simulink model "lab2_floating_01slx"  (R2022a)
settings: Solver=VariableStepAuto  StartTime=0.0  StopTime=10.0  RelTol=1e-3
settings Model: Creator=Illia  LastModifiedBy=Illia

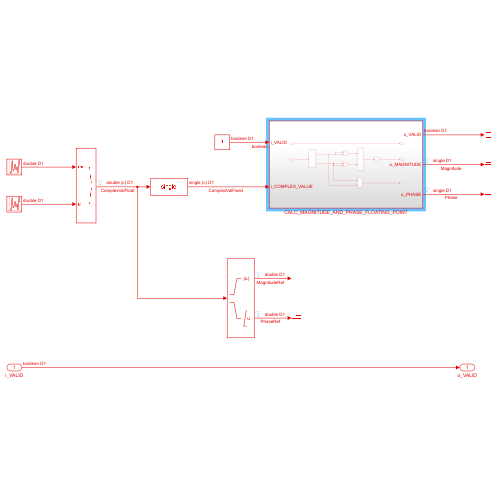
[thumbnail: Simulink's stored preview of the top-level diagram]
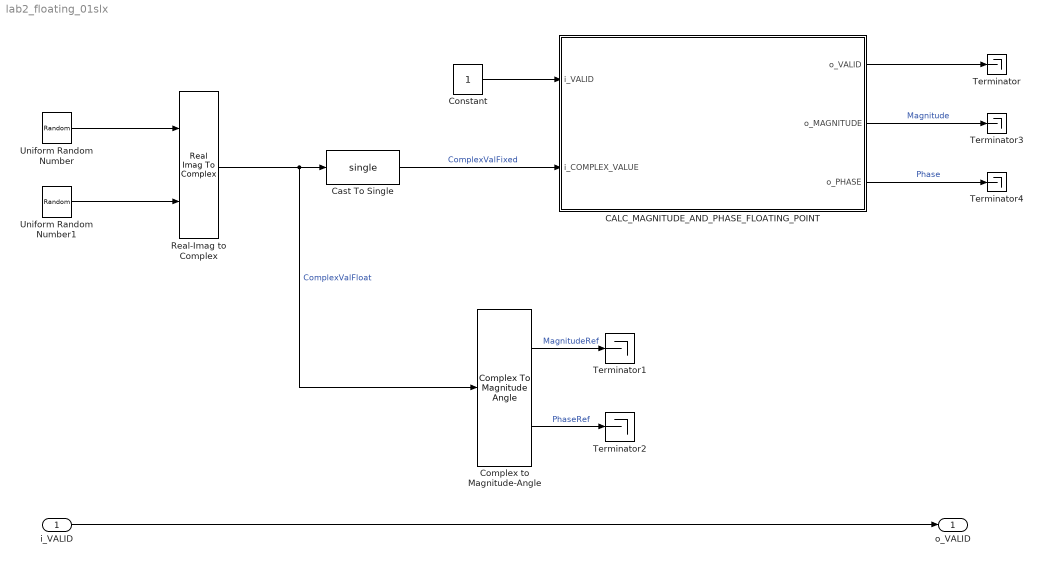
== system lab2_floating_01slx ==
  i_VALID : Inport  OutDataTypeStr=boolean
  CALC_MAGNITUDE_AND_PHASE_FLOATING_POINT : Subsystem
  Cast To Single : DataTypeConversion  OutDataTypeStr=single  RndMeth=Nearest  SaturateOnIntegerOverflow=off
  Complex to Magnitude-Angle : ComplexToMagnitudeAngle
  Constant : Constant  OutDataTypeStr=boolean  SampleTime=1
  Real-Imag to Complex : RealImagToComplex
  Terminator{,1..4} (5 alike) : Terminator
  Uniform Random Number : UniformRandomNumber  Minimum=-4  Maximum=4  Seed=5  SampleTime=1
  Uniform Random Number1 : UniformRandomNumber  Seed=6  SampleTime=1
  o_VALID : Outport  VectorParamsAs1DForOutWhenUnconnected=off
  wires:
  i_VALID/1 -> o_VALID/1
  Cast To Single/1 -> CALC_MAGNITUDE_AND_PHASE_FLOATING_POINT/2(i_COMPLEX_VALUE)  "ComplexValFixed"
  Constant/1 -> CALC_MAGNITUDE_AND_PHASE_FLOATING_POINT/1(i_VALID)
  CALC_MAGNITUDE_AND_PHASE_FLOATING_POINT/3(o_PHASE) -> Terminator4/1  "Phase"
  Complex to Magnitude-Angle/2 -> Terminator2/1  "PhaseRef"
  CALC_MAGNITUDE_AND_PHASE_FLOATING_POINT/2(o_MAGNITUDE) -> Terminator3/1  "Magnitude"
  Real-Imag to Complex/1 -> Cast To Single/1, Complex to Magnitude-Angle/1  "ComplexValFloat"
  Uniform Random Number/1 -> Real-Imag to Complex/1
  Complex to Magnitude-Angle/1 -> Terminator1/1  "MagnitudeRef"
  Uniform Random Number1/1 -> Real-Imag to Complex/2
  CALC_MAGNITUDE_AND_PHASE_FLOATING_POINT/1(o_VALID) -> Terminator/1

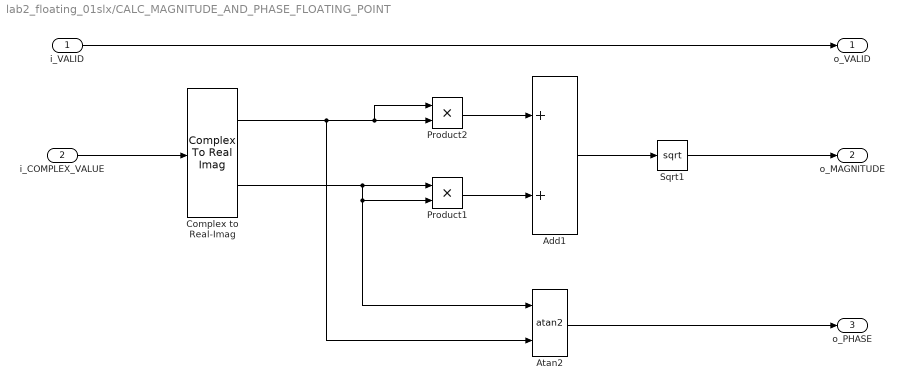
== system lab2_floating_01slx/CALC_MAGNITUDE_AND_PHASE_FLOATING_POINT ==
  i_VALID : Inport  OutDataTypeStr=boolean
  i_COMPLEX_VALUE : Inport  Port=2
  Add1 : Sum
  Atan2 : Trigonometry  Operator=atan2
  Complex to Real-Imag : ComplexToRealImag
  Product1 : Product
  Product2 : Product
  Sqrt1 : Sqrt  OutDataTypeStr=Inherit: Inherit via internal rule
  o_VALID : Outport  VectorParamsAs1DForOutWhenUnconnected=off
  o_MAGNITUDE : Outport  Port=2
  o_PHASE : Outport  Port=3
  wires:
  i_COMPLEX_VALUE/1 -> Complex to Real-Imag/1
  i_VALID/1 -> o_VALID/1
  Complex to Real-Imag/1 -> Atan2/2, Product2/1, Product2/2
  Complex to Real-Imag/2 -> Product1/1, Product1/2, Atan2/1
  Product1/1 -> Add1/2
  Product2/1 -> Add1/1
  Add1/1 -> Sqrt1/1
  Sqrt1/1 -> o_MAGNITUDE/1
  Atan2/1 -> o_PHASE/1
